simulink model "ZT_VehCtrl_18B"  (R2018b)
settings: Solver=FixedStepAuto  StartTime=0.0  StopTime=inf  FixedStep=0.005  RelTol=1e-3
InitFcn:
  | mbd_mpc_consistency_checks(bdroot(gcs));
undefined symbols (not defined in the file): ANG_DEAD, BMS_NormalPwr, BrkPrsByBrkPct_TB_X, BrkPrsByBrkPct_TB_Y, DELAY_DISCHARGE, DELAY_RCUOFF, DRV_BACKWARD, DRV_BRAKE, DRV_FORWARD, DRV_NEUTRAL, DRV_PARK, DRV_UNPARK, DRV_ZEROTURN, EPB_LOCK, EPB_UNLOCK, ExtraLoadPwr, FanOff, fifo_0_vect, fifo_1_vect, HiFanReq, HV_finished, HV_No_Active, HV_POWER_OFF, HV_POWER_ON, HVDown, HVON, KaTLS_v_DrgUp_X_VehSpd, KeFTM_s_Way1OffDlyTime, KeFTM_TK_Way1CoolLv2OffBatTemp, KeFTM_TK_Way1CoolLv2OffMtrTemp, KeFTM_TK_Way1CoolLv2OnBatTemp, KeFTM_TK_Way1CoolLv2OnMtrTemp, KeFTM_TK_Way1CoolLv3OffBatTemp, KeFTM_TK_Way1CoolLv3OffMtrTemp, KeFTM_TK_Way1CoolLv3OnBatTemp, KeFTM_TK_Way1CoolLv3OnMtrTemp, KeFTM_TK_Way1CoolLv4OffBatTemp, KeFTM_TK_Way1CoolLv4OffMtrTemp, KeFTM_TK_Way1CoolLv4OnBatTemp, KeFTM_TK_Way1CoolLv4OnMtrTemp, Kp1, Kp2, LowFanReq, LQFP, MtrPwrFactor_RCU, MtrPwrHighToMidThd, MtrPwrLowToMidThd, MtrPwrMidToHighThd, MtrPwrMidToLowThd, MtrTrqMax, PCT_DEAD, Precharge, PTO_1000, PTO_540, pts1_fifo_0_vect, pts1_fifo_1_vect, pts2_fifo_0_vect, pts2_fifo_1_vect, pts3_fifo_0_vect, pts3_fifo_1_vect ... (+24)
libraries: mbd_mpc574x_ec_toolbox x124, canmsglib x72, simulink x57
(part 4 of 11)

== system ZT_VehCtrl_18B/VehCtrl/EnergyManage1 ==
  DriverIn : Inport
  VehTrqTgt : Inport  Port=2
  VehSpd : Inport  Port=3
  RCU : Inport  Port=4
  Fault : Inport  Port=5
  MCU_PTO : Inport  Port=6
  BMS : Inport  Port=7
  "RMT " : Inport  Port=8
  MtrPwrOutTotal : Inport  Port=9
  Add : Sum
  Bus Creator1 : BusCreator  Inputs=7
  Bus Creator2 : BusCreator  Inputs=2
  Bus Creator3 : BusCreator  Inputs=1
  Bus Creator4 : BusCreator  Inputs=1
  Bus Selector : BusSelector  OutputSignals=KeyStatus
  Bus Selector1 : BusSelector  OutputSignals=ShutDown
  Bus Selector2 : BusSelector  OutputSignals=OBC_Charger Status.RCU_RexSelfChkSt,OBC_Charger Status.RCU_RexFltLvl,BMS_Charger Status.RCU_RexGenPwrMaxLim,RCU_MSG_3.RCU_GCUISGInverterTempHiAlarm,RCU_MSG_3.RCU_GCUISGMotorTempHiAlarm
  Bus Selector3 : BusSelector  OutputSignals=RMT4.RMT_RCU
  Bus Selector4 : BusSelector  OutputSignals=BMS Power Infor.APPSOC,BMS_PackStateInf.BMS_BatteryState,BMS_Relay Status.IPI_ChrgSignal,BMS_Relay Status.IPI_CC2St
  Chart : Stateflow chart  TreatAsAtomicUnit=on
  Chart1 : Stateflow chart  TreatAsAtomicUnit=on
  Constant : Constant  Value=ExtraLoadPwr
  Data Store Write : DataStoreWrite  DataStoreName=Flag
  Logical Operator : Logic  Operator=OR  AllPortsSameDT=off  OutDataTypeStr=boolean
  Subsystem : Subsystem
  BMS_OUT : Outport
  RCU_OUT : Outport  Port=2
  DCDC_OUT : Outport  Port=3
  MCU_COM : Outport  Port=4
  Ready : Outport  Port=5
  EN_COM : Outport  Port=6
  wires:
  Add/1 -> Chart1/1(MtrPwrTotal)
  Chart/7(VCU_MotwaterPumpDutyRe) -> Bus Creator1/6  "VCU_MotwaterPumpDutyRe"
  Constant/1 -> Add/2
  MtrPwrOutTotal/1 -> Add/1
  Chart1/1(RCU_RexGenPwr) -> Chart/13(RCU_RexGenPwr)
  Bus Selector4/1 -> Chart/9(BMS_SOC)  "<APPSOC>"
  Bus Selector2/1 -> Chart/3(RCU_RexSelfChkSt)  "<RCU_RexSelfChkSt>"
  Chart/13(Flag) -> Data Store Write/1
  Chart/1(VCU_Maincircuitcommand) -> Bus Creator4/1  "VCU_Maincircuitcommand"
  Chart/3(VCU_RexEnableCmd) -> Bus Creator1/2  "VCU_RexEnableCmd"
  "RMT "/1 -> Bus Selector3/1
  VehSpd/1 -> Subsystem/2(VehSpd)
  Bus Creator2/1 -> MCU_COM/1
  Bus Selector4/3 -> Logical Operator/1  "<IPI_ChrgSignal>"
  Chart/8(VCU_RexActiveDischgCmd) -> Bus Creator1/7  "VCU_RexActiveDischgCmd"
  VehTrqTgt/1 -> Subsystem/1(VehTrqTgt)
  Bus Selector3/1 -> Chart/12(Rcuswitch)  "<RMT_RCU>"
  Bus Selector4/4 -> Logical Operator/2  "<IPI_CC2St>"
  Chart/11(Ready) -> Ready/1  "Ready"
  Bus Selector2/5 -> Chart/7(RCU_GCUISGMotorTempHiAlarm)  "<RCU_GCUISGMotorTempHiAlarm>"
  Chart/6(VCU_FanStsReg) -> Bus Creator1/5  "VCU_FanStsReg"
  Bus Selector2/4 -> Chart/6(RCU_GCUISGInverterTempHiAlarm)  "<RCU_GCUISGInverterTempHiAlarm>"
  Bus Creator3/1 -> DCDC_OUT/1
  Bus Creator4/1 -> BMS_OUT/1
  Bus Selector/1 -> Chart/1(Key)  "<KeyStatus>"
  Chart/12(DCDC_Enable) -> Bus Creator3/1  "DCDC_Enable"
  Chart/10(MCU_Discharge) -> Bus Creator2/2  "MCU_Discharge"
  Bus Selector2/3 -> Chart/5(RCU_RexGenPwrMaxLim)  "<RCU_RexGenPwrMaxLim>"
  Chart/4(VCU_RexStartStopReq) -> Bus Creator1/3  "VCU_RexStartStopReq"
  Bus Creator1/1 -> RCU_OUT/1
  Subsystem/1(PwrCmd) -> Chart/8(MCU_TotalPwrCmd)
  Chart/2(VCU_HVOnOffSts) -> Bus Creator1/1  "VCU_HVOnOffSts"
  DriverIn/1 -> Bus Selector/1
  RCU/1 -> Bus Selector2/1
  Bus Selector2/2 -> Chart/4(RCU_RexFltLvl)  "<RCU_RexFltLvl>"
  Bus Selector4/2 -> Chart/10(BMS_BatteryState)  "<BMS_BatteryState>"
  Fault/1 -> Bus Selector1/1
  BMS/1 -> Bus Selector4/1
  MCU_PTO/1 -> Subsystem/3(MCU_PTO)
  Chart/5(VCU_ReqRexGenPwr) -> Bus Creator1/4  "VCU_ReqRexGenPwr"
  Logical Operator/1 -> Chart/11(ChrgSig)
  Chart/9(MCU_Enable) -> Bus Creator2/1, EN_COM/1  "MCU_Enable"
  Bus Selector1/1 -> Chart/2(ShutDown)  "<ShutDown>"

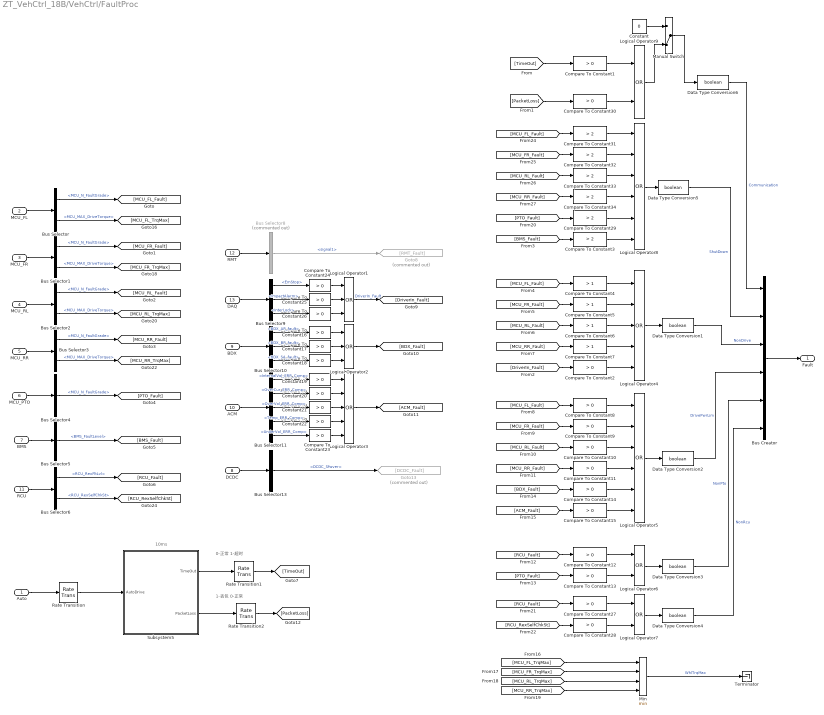
== system ZT_VehCtrl_18B/VehCtrl/FaultProc ==
  note: 10ms
  note: 0-正常
      | 1-超时
  note: 1-丢包
      | 0-正常
  Auto : Inport
  MCU_FL : Inport  Port=2
  MCU_FR : Inport  Port=3
  MCU_RL : Inport  Port=4
  MCU_RR : Inport  Port=5
  MCU_PTO : Inport  Port=6
  BMS : Inport  Port=7
  DCDC : Inport  Port=8
  BDX : Inport  Port=9
  ACM : Inport  Port=10
  RCU : Inport  Port=11
  RMT : Inport  Port=12
  DAQ : Inport  Port=13
  Bus Creator : BusCreator  Inputs=6
  Bus Selector{,1..3} (4 alike) : BusSelector  OutputSignals=MCU2VCU_3.MCU_N_FaultGrade,MCU2VCU_4.MCU_MAX_DriveTorque
  Bus Selector10 : BusSelector  OutputSignals=AVCU.BDX_AP_fault,AVCU.BDX_BP_fault,AVCU.BDX_SA_fault
  Bus Selector11 : BusSelector  OutputSignals=InternalVol_ERR_Comp,OverCur_ERR_Comp,OverVol_ERR_Comp,Temp_ERR_Comp,UnderVol_ERR_Comp
  Bus Selector13 : BusSelector  OutputSignals=DCDC_Sfwver
  Bus Selector4 : BusSelector  OutputSignals=MCU2VCU_3.MCU_N_FaultGrade
  Bus Selector5 : BusSelector  OutputSignals=BMS_PackStateInf.BMS_FaultLevel
  Bus Selector6 : BusSelector  OutputSignals=OBC_Charger Status.RCU_RexFltLvl,OBC_Charger Status.RCU_RexSelfChkSt
  Bus Selector8 : BusSelector  Commented=on  OutputSignals=RMT3.signal1
  Bus Selector9 : BusSelector  OutputSignals=EmStop,ImpactAlarm,InterLock
  Compare To Constant{1..2,8..28,30} (24 alike) : simulink/Logic and Bit Operations/Compare To Constant  relop=>  const=0  OutDataTypeStr=boolean
  Compare To Constant{3,29,31..34} (6 alike) : simulink/Logic and Bit Operations/Compare To Constant  relop=>  const=2  OutDataTypeStr=boolean
  Compare To Constant{4..7} (4 alike) : simulink/Logic and Bit Operations/Compare To Constant  relop=>  const=1  OutDataTypeStr=boolean
  Constant : Constant  Value=0
  Data Type Conversion{1..6} (6 alike) : DataTypeConversion  OutDataTypeStr=boolean
  Goto13 : Goto  Commented=on  GotoTag=DCDC_Fault
  Goto8 : Goto  Commented=on  GotoTag=RMT_Fault
  Logical Operator1 : Logic  Operator=OR  Inputs=3  AllPortsSameDT=off  OutDataTypeStr=boolean
  Logical Operator2 : Logic  Operator=OR  Inputs=3  AllPortsSameDT=off  OutDataTypeStr=boolean
  Logical Operator3 : Logic  Operator=OR  Inputs=5  AllPortsSameDT=off  OutDataTypeStr=boolean
  Logical Operator4 : Logic  Operator=OR  Inputs=5  AllPortsSameDT=off  OutDataTypeStr=boolean
  Logical Operator5 : Logic  Operator=OR  Inputs=6  AllPortsSameDT=off  OutDataTypeStr=boolean
  Logical Operator6 : Logic  Operator=OR  AllPortsSameDT=off  OutDataTypeStr=boolean
  Logical Operator7 : Logic  Operator=OR  AllPortsSameDT=off  OutDataTypeStr=boolean
  Logical Operator8 : Logic  Operator=OR  Inputs=6  AllPortsSameDT=off  OutDataTypeStr=boolean
  Logical Operator9 : Logic  Operator=OR  AllPortsSameDT=off  OutDataTypeStr=boolean
  Manual Switch : ManualSwitch  CurrentSetting=0
  Min : MinMax  Inputs=4
  Rate Transition : RateTransition
  Rate Transition1 : RateTransition
  Rate Transition2 : RateTransition
  Subsystem5 : Subsystem  TreatAsAtomicUnit=on  SystemSampleTime=0.01
  Terminator : Terminator
  Fault : Outport
  wires:
  Logical Operator8/1 -> Data Type Conversion5/1
  Data Type Conversion1/1 -> Bus Creator/3  "NonDrive"
  Data Type Conversion2/1 -> Bus Creator/4  "DrivePwrLim"
  Data Type Conversion3/1 -> Bus Creator/5  "NonPto"
  Bus Creator/1 -> Fault/1
  MCU_FL/1 -> Bus Selector/1
  Bus Selector/1 -> [MCU_FL_Fault]  "<MCU_N_FaultGrade>"
  Bus Selector1/1 -> [MCU_FR_Fault]  "<MCU_N_FaultGrade>"
  MCU_FR/1 -> Bus Selector1/1
  MCU_RR/1 -> Bus Selector3/1
  Bus Selector3/1 -> [MCU_RR_Fault]  "<MCU_N_FaultGrade>"
  Bus Selector2/1 -> [MCU_RL_Fault]  "<MCU_N_FaultGrade>"
  MCU_RL/1 -> Bus Selector2/1
  Bus Selector4/1 -> [PTO_Fault]  "<MCU_N_FaultGrade>"
  MCU_PTO/1 -> Bus Selector4/1
  BMS/1 -> Bus Selector5/1
  Bus Selector5/1 -> [BMS_Fault]  "<BMS_FaultLevel>"
  Bus Selector6/1 -> [RCU_Fault]  "<RCU_RexFltLvl>"
  RCU/1 -> Bus Selector6/1
  Bus Selector8/1 -> Goto8/1  "<signal1>"
  RMT/1 -> Bus Selector8/1
  DAQ/1 -> Bus Selector9/1
  Bus Selector9/1 -> Compare To Constant24/1  "<EmStop>"
  Bus Selector9/2 -> Compare To Constant25/1  "<ImpactAlarm>"
  Bus Selector9/3 -> Compare To Constant26/1  "<InterLock>"
  Logical Operator1/1 -> [DriverIn_Fault]  "DriverIn_Fault"
  BDX/1 -> Bus Selector10/1
  Logical Operator2/1 -> [BDX_Fault]
  Bus Selector10/3 -> Compare To Constant18/1  "<BDX_SA_fault>"
  Bus Selector10/2 -> Compare To Constant17/1  "<BDX_BP_fault>"
  Bus Selector10/1 -> Compare To Constant16/1  "<BDX_AP_fault>"
  ACM/1 -> Bus Selector11/1
  Bus Selector11/1 -> Compare To Constant19/1  "<InternalVol_ERR_Comp>"
  Bus Selector11/2 -> Compare To Constant20/1  "<OverCur_ERR_Comp>"
  Bus Selector11/3 -> Compare To Constant21/1  "<OverVol_ERR_Comp>"
  Logical Operator3/1 -> [ACM_Fault]
  Bus Selector11/4 -> Compare To Constant22/1  "<Temp_ERR_Comp>"
  Bus Selector11/5 -> Compare To Constant23/1  "<UnderVol_ERR_Comp>"
  DCDC/1 -> Bus Selector13/1
  Bus Selector13/1 -> Goto13/1  "<DCDC_Sfwver>"
  [DriverIn_Fault] -> Compare To Constant2/1
  [BMS_Fault] -> Compare To Constant3/1
  Logical Operator4/1 -> Data Type Conversion1/1
  [MCU_FL_Fault] -> Compare To Constant4/1
  Compare To Constant4/1 -> Logical Operator4/1
  Compare To Constant5/1 -> Logical Operator4/2
  [MCU_FR_Fault] -> Compare To Constant5/1
  [MCU_RR_Fault] -> Compare To Constant7/1
  Compare To Constant7/1 -> Logical Operator4/4
  Compare To Constant6/1 -> Logical Operator4/3
  [MCU_RL_Fault] -> Compare To Constant6/1
  Logical Operator5/1 -> Data Type Conversion2/1
  [MCU_RL_Fault] -> Compare To Constant10/1
  Compare To Constant10/1 -> Logical Operator5/3
  Compare To Constant11/1 -> Logical Operator5/4
  [MCU_RR_Fault] -> Compare To Constant11/1
  [MCU_FR_Fault] -> Compare To Constant9/1
  Compare To Constant9/1 -> Logical Operator5/2
  Compare To Constant8/1 -> Logical Operator5/1
  [MCU_FL_Fault] -> Compare To Constant8/1
  Logical Operator6/1 -> Data Type Conversion3/1
  [RCU_Fault] -> Compare To Constant12/1
  Compare To Constant12/1 -> Logical Operator6/1
  Compare To Constant13/1 -> Logical Operator6/2
  [PTO_Fault] -> Compare To Constant13/1
  [BDX_Fault] -> Compare To Constant14/1
  Compare To Constant14/1 -> Logical Operator5/5
  Compare To Constant15/1 -> Logical Operator5/6
  [ACM_Fault] -> Compare To Constant15/1
  Bus Selector/2 -> [MCU_FL_TrqMax]  "<MCU_MAX_DriveTorque>"
  Bus Selector1/2 -> [MCU_FR_TrqMax]  "<MCU_MAX_DriveTorque>"
  Bus Selector2/2 -> [MCU_RL_TrqMax]  "<MCU_MAX_DriveTorque>"
  Bus Selector3/2 -> [MCU_RR_TrqMax]  "<MCU_MAX_DriveTorque>"
  [MCU_FL_TrqMax] -> Min/1
  [MCU_FR_TrqMax] -> Min/2
  [MCU_RL_TrqMax] -> Min/3
  [MCU_RR_TrqMax] -> Min/4
  Compare To Constant16/1 -> Logical Operator2/1
  Compare To Constant17/1 -> Logical Operator2/2
  Compare To Constant18/1 -> Logical Operator2/3
  Compare To Constant19/1 -> Logical Operator3/1
  Compare To Constant20/1 -> Logical Operator3/2
  Compare To Constant21/1 -> Logical Operator3/3
  Compare To Constant22/1 -> Logical Operator3/4
  Compare To Constant23/1 -> Logical Operator3/5
  Compare To Constant24/1 -> Logical Operator1/1
  Compare To Constant25/1 -> Logical Operator1/2
  Compare To Constant26/1 -> Logical Operator1/3
  Bus Selector6/2 -> [RCU_RexSelfChkSt]  "<RCU_RexSelfChkSt>"
  [RCU_RexSelfChkSt] -> Compare To Constant28/1
  Compare To Constant28/1 -> Logical Operator7/2
  Compare To Constant27/1 -> Logical Operator7/1
  [RCU_Fault] -> Compare To Constant27/1
  Logical Operator7/1 -> Data Type Conversion4/1
  Data Type Conversion4/1 -> Bus Creator/6  "NonRcu"
  Compare To Constant2/1 -> Logical Operator4/5
  [MCU_RL_Fault] -> Compare To Constant33/1
  Compare To Constant33/1 -> Logical Operator8/3
  Compare To Constant34/1 -> Logical Operator8/4
  [MCU_RR_Fault] -> Compare To Constant34/1
  [MCU_FR_Fault] -> Compare To Constant32/1
  Compare To Constant32/1 -> Logical Operator8/2
  Compare To Constant31/1 -> Logical Operator8/1
  [MCU_FL_Fault] -> Compare To Constant31/1
  Compare To Constant3/1 -> Logical Operator8/6
  [PTO_Fault] -> Compare To Constant29/1
  Compare To Constant29/1 -> Logical Operator8/5
  Min/1 -> Terminator/1  "WhlTrqMax"
  Rate Transition1/1 -> [TimeOut]
  Auto/1 -> Rate Transition/1
  Subsystem5/2(PacketLoss) -> Rate Transition2/1
  Rate Transition/1 -> Subsystem5/1(AutoDrive)
  Rate Transition2/1 -> [PacketLoss]
  Subsystem5/1(TimeOut) -> Rate Transition1/1
  Data Type Conversion5/1 -> Bus Creator/2  "ShutDown"
  [TimeOut] -> Compare To Constant1/1
  [PacketLoss] -> Compare To Constant30/1
  Compare To Constant1/1 -> Logical Operator9/1
  Compare To Constant30/1 -> Logical Operator9/2
  Manual Switch/1 -> Data Type Conversion6/1
  Data Type Conversion6/1 -> Bus Creator/1  "Communication"
  Constant/1 -> Manual Switch/1
  Logical Operator9/1 -> Manual Switch/2

== system ZT_VehCtrl_18B/VehCtrl/LedControl ==
  note: LS015-红灯
      | LS016-绿灯
      | 都亮为黄灯
  BMS : Inport
  cmd : Inport  Port=2
  Bus Selector : BusSelector  OutputSignals=StrAng,BrkPct,ModeDir
  Bus Selector1 : BusSelector  OutputSignals=BMS_PackStateInf.BMS_BatteryState,BMS Power Infor.APPSOC
  Chart : Stateflow chart  TreatAsAtomicUnit=on
  Chart1 : Stateflow chart  TreatAsAtomicUnit=on
  Compare To Constant : simulink/Logic and Bit Operations/Compare To Constant  relop===  const=3.0  OutDataTypeStr=boolean
  Constant : Constant  Value=0  OutDataTypeStr=boolean
  Constant1 : Constant  OutDataTypeStr=boolean
  Data Store Read : DataStoreRead  DataStoreName=Fault
  Data Store Read1 : DataStoreRead  DataStoreName=CtrMode
  Data Store Write : DataStoreWrite  DataStoreName=HS002
  Data Store Write1 : DataStoreWrite  DataStoreName=HS003
  Data Store Write2 : DataStoreWrite  DataStoreName=HS005
  Data Store Write3 : DataStoreWrite  DataStoreName=HS007
  Data Store Write4 : DataStoreWrite  DataStoreName=HS010
  Data Store Write5 : DataStoreWrite  DataStoreName=LS015
  Data Store Write6 : DataStoreWrite  DataStoreName=LS016
  Data Type Conversion{,1..3} (4 alike) : DataTypeConversion  OutDataTypeStr=boolean
  Data Type Conversion{4..7} (4 alike) : DataTypeConversion
  Switch : Switch  Threshold=1
  wires:
  cmd/1 -> Bus Selector/1
  Bus Selector/1 -> Chart/2(SteerAng)  "<StrAng>"
  Chart/1(Left_Cmd) -> Data Type Conversion1/1
  Chart/2(Right_Cmd) -> Data Type Conversion2/1
  Bus Selector/2 -> Switch/2  "<BrkPct>"
  Bus Selector/3 -> Data Type Conversion/1  "<ModeDir>"
  Data Type Conversion1/1 -> Data Store Write1/1
  Data Type Conversion2/1 -> Data Store Write/1
  Switch/1 -> Data Store Write3/1
  Data Type Conversion/1 -> Data Store Write4/1
  Constant1/1 -> Switch/1
  Constant/1 -> Switch/3
  BMS/1 -> Bus Selector1/1
  Bus Selector1/2 -> Chart/1(soc)  "<APPSOC>"
  Data Type Conversion3/1 -> Data Store Write2/1
  Compare To Constant/1 -> Data Type Conversion3/1
  Bus Selector1/1 -> Compare To Constant/1  "<BMS_BatteryState>"
  Chart1/1(Red) -> Data Type Conversion4/1
  Chart1/2(Green) -> Data Type Conversion5/1
  Data Store Read1/1 -> Data Type Conversion6/1
  Data Store Read/1 -> Data Type Conversion7/1
  Data Type Conversion4/1 -> Data Store Write5/1
  Data Type Conversion5/1 -> Data Store Write6/1
  Data Type Conversion6/1 -> Chart1/1(CtrMode)
  Data Type Conversion7/1 -> Chart1/2(Fault)

== system ZT_VehCtrl_18B/VehCtrl/MontionControl ==
  EN_COM : Inport
  Ready : Inport  Port=2
  CMD : Inport  Port=3
  VehSpd : Inport  Port=4
  BDX : Inport  Port=5
  Fault : Inport  Port=6
  AUTOMode : Inport  Port=7
  AUTO : Inport  Port=8
  BMS : Inport  Port=9
  RMT : Inport  Port=10
  DCDC : Inport  Port=11
  DriveControl : Subsystem
  PtoControl : Subsystem
  SteerControl : Subsystem
  ValveControl : Subsystem
  MCUFL_OUT : Outport
  MCUFR_OUT : Outport  Port=2
  MCURL_OUT : Outport  Port=3
  MCURR_OUT : Outport  Port=4
  MCU_PTO_OUT : Outport  Port=5
  BDX_OUT : Outport  Port=6
  VehTrqTgt : Outport  Port=7
  wires:
  CMD/1 -> PtoControl/1(CMD), ValveControl/4(CMD), SteerControl/2(CMD), DriveControl/4(CMD)
  BDX/1 -> ValveControl/3(BDX), SteerControl/3(BDX)
  SteerControl/1(StrReady) -> DriveControl/7(StrReady)
  VehSpd/1 -> ValveControl/8(VehSpd), SteerControl/1(VehSpd), DriveControl/6(VehSpd)
  DriveControl/5(BrkPrsTgt) -> ValveControl/1(BrkPrsTgt)
  DriveControl/6(EpbSt) -> ValveControl/2(EpbSt)
  DriveControl/1(MCUFL_OUT) -> MCUFL_OUT/1
  DriveControl/2(MCUFR_OUT) -> MCUFR_OUT/1
  DriveControl/4(MCURR_OUT) -> MCURR_OUT/1
  DriveControl/3(MCURL_OUT) -> MCURL_OUT/1
  ValveControl/1(BDX_OUT) -> BDX_OUT/1
  Ready/1 -> PtoControl/3(Ready), ValveControl/5(Ready), DriveControl/2(Ready)
  PtoControl/1(MCU_PTO_OUT) -> MCU_PTO_OUT/1
  DriveControl/7(VehTrqTgt) -> VehTrqTgt/1
  SteerControl/2(AngCmd) -> ValveControl/6("AngCmd ")
  AUTOMode/1 -> PtoControl/4(AUTOMode), DriveControl/9(AUTOMode)
  AUTO/1 -> PtoControl/5(AUTO), DriveControl/8(AUTO)
  BMS/1 -> DriveControl/5(BMS)
  RMT/1 -> DriveControl/10(RMT)
  DCDC/1 -> DriveControl/11(DCDC)
  Fault/1 -> PtoControl/2(Fault), ValveControl/7(fault), DriveControl/3(Fault)
  EN_COM/1 -> DriveControl/1(EN_COM)

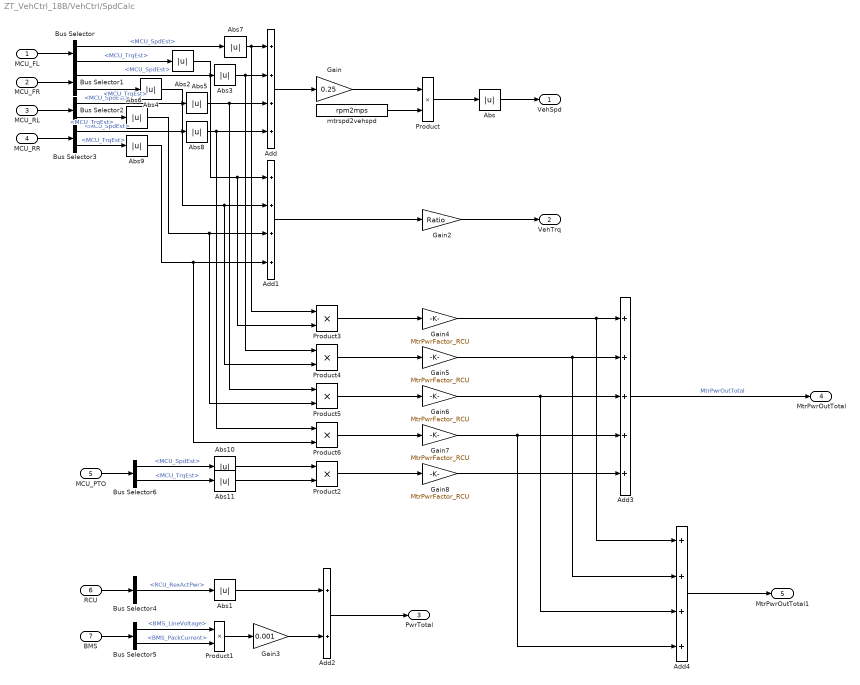
== system ZT_VehCtrl_18B/VehCtrl/SpdCalc ==
  MCU_FL : Inport
  MCU_FR : Inport  Port=2
  MCU_RL : Inport  Port=3
  MCU_RR : Inport  Port=4
  MCU_PTO : Inport  Port=5
  RCU : Inport  Port=6
  BMS : Inport  Port=7
  Abs{,1..11} (12 alike) : Abs
  Add : Sum  Inputs=++++
  Add1 : Sum  Inputs=++++
  Add2 : Sum
  Add3 : Sum  Inputs=+++++
  Add4 : Sum  Inputs=4
  Bus Selector{,1..3,6} (5 alike) : BusSelector  OutputSignals=MCU2VCU_1.MCU_SpdEst,MCU2VCU_1.MCU_TrqEst
  Bus Selector4 : BusSelector  OutputSignals=BMS_Charger Status.RCU_RexActPwr
  Bus Selector5 : BusSelector  OutputSignals=BMS_PackMeasure.BMS_LineVoltage,BMS_PackMeasure.BMS_PackCurrent
  Gain : Gain  Gain=0.25
  Gain2 : Gain  Gain=Ratio
  Gain3 : Gain  Gain=0.001
  Gain{4..8} (5 alike) : Gain  Gain=MtrPwrFactor_RCU
  Product{,1..6} (7 alike) : Product
  mtrspd2vehspd : Constant  Value=rpm2mps
  VehSpd : Outport
  "VehTrq " : Outport  Port=2
  PwrTotal : Outport  Port=3
  MtrPwrOutTotal : Outport  Port=4
  MtrPwrOutTotal1 : Outport  Port=5
  wires:
  Add/1 -> Gain/1
  Gain/1 -> Product/1
  Product/1 -> Abs/1
  mtrspd2vehspd/1 -> Product/2
  MCU_FL/1 -> Bus Selector/1
  Bus Selector/1 -> Abs7/1  "<MCU_SpdEst>"
  Bus Selector1/1 -> Abs3/1  "<MCU_SpdEst>"
  MCU_FR/1 -> Bus Selector1/1
  MCU_RR/1 -> Bus Selector3/1
  Bus Selector3/1 -> Abs8/1  "<MCU_SpdEst>"
  Bus Selector2/1 -> Abs5/1  "<MCU_SpdEst>"
  MCU_RL/1 -> Bus Selector2/1
  Abs/1 -> VehSpd/1
  Bus Selector/2 -> Abs2/1  "<MCU_TrqEst>"
  Bus Selector1/2 -> Abs4/1  "<MCU_TrqEst>"
  Bus Selector2/2 -> Abs6/1  "<MCU_TrqEst>"
  Bus Selector3/2 -> Abs9/1  "<MCU_TrqEst>"
  Add1/1 -> Gain2/1
  Gain2/1 -> "VehTrq "/1
  RCU/1 -> Bus Selector4/1
  BMS/1 -> Bus Selector5/1
  Bus Selector5/1 -> Product1/1  "<BMS_LineVoltage>"
  Bus Selector5/2 -> Product1/2  "<BMS_PackCurrent>"
  Product1/1 -> Gain3/1
  Bus Selector4/1 -> Abs1/1  "<RCU_RexActPwr>"
  Gain3/1 -> Add2/2
  Abs1/1 -> Add2/1
  Add2/1 -> PwrTotal/1
  MCU_PTO/1 -> Bus Selector6/1
  Bus Selector6/1 -> Abs10/1  "<MCU_SpdEst>"
  Bus Selector6/2 -> Abs11/1  "<MCU_TrqEst>"
  Product3/1 -> Gain4/1
  Product2/1 -> Gain8/1
  Product6/1 -> Gain7/1
  Product5/1 -> Gain6/1
  Product4/1 -> Gain5/1
  Gain4/1 -> Add4/1, Add3/1
  Gain5/1 -> Add4/2, Add3/2
  Gain6/1 -> Add4/3, Add3/3
  Gain8/1 -> Add3/5
  Add3/1 -> MtrPwrOutTotal/1  "MtrPwrOutTotal"
  Gain7/1 -> Add4/4, Add3/4
  Abs7/1 -> Product3/1, Add/1
  Abs2/1 -> Product3/2, Add1/1
  Abs3/1 -> Product4/1, Add/2
  Abs4/1 -> Product4/2, Add1/2
  Abs5/1 -> Product5/1, Add/3
  Abs6/1 -> Product5/2, Add1/3
  Abs8/1 -> Product6/1, Add/4
  Abs9/1 -> Product6/2, Add1/4
  Abs10/1 -> Product2/1
  Abs11/1 -> Product2/2
  Add4/1 -> MtrPwrOutTotal1/1

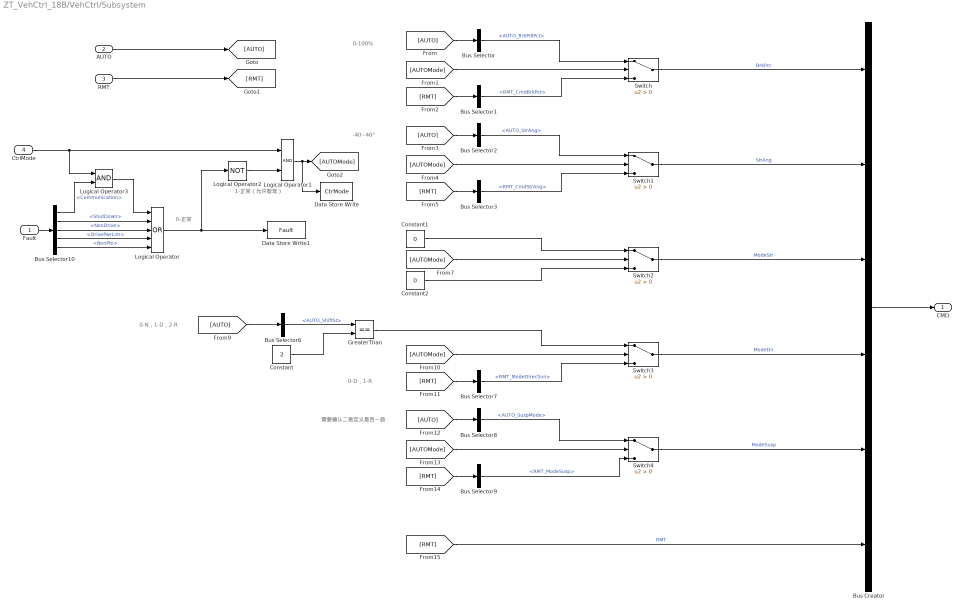
== system ZT_VehCtrl_18B/VehCtrl/Subsystem ==
  note: 0-正常
  note: -40~40°
  note: 0-100%
  note: 0-N，1-D，2-R
  note: 0-D，1-R
  note: 需要确认二者定义是否一致
  note: 1-正常（允许智驾）
  Fault : Inport
  AUTO : Inport  Port=2
  RMT : Inport  Port=3
  CtrlMode : Inport  Port=4
  Bus Creator : BusCreator  Inputs=6
  Bus Selector : BusSelector  OutputSignals=signal1.AUTO_BrkPdlPct
  Bus Selector1 : BusSelector  OutputSignals=RMT1.RMT_CmdBrkPct
  Bus Selector10 : BusSelector  OutputSignals=Communication,ShutDown,NonDrive,DrivePwrLim,NonPto
  Bus Selector2 : BusSelector  OutputSignals=signal1.AUTO_StrAng
  Bus Selector3 : BusSelector  OutputSignals=RMT1.RMT_CmdStrAng
  Bus Selector6 : BusSelector  OutputSignals=signal1.AUTO_ShiftSt
  Bus Selector7 : BusSelector  OutputSignals=RMT3.RMT_ModeDirection
  Bus Selector8 : BusSelector  OutputSignals=signal2.AUTO_SuspMode
  Bus Selector9 : BusSelector  OutputSignals=RMT2.RMT_ModeSusp
  Constant : Constant  Value=2  OutDataTypeStr=uint8
  Constant1 : Constant  Value=0  OutDataTypeStr=boolean
  Constant2 : Constant  Value=0  OutDataTypeStr=boolean
  Data Store Write : DataStoreWrite  DataStoreName=CtrMode
  Data Store Write1 : DataStoreWrite  DataStoreName=Fault
  GreaterThan : RelationalOperator  Operator===  OutDataTypeStr=boolean  RndMeth=Simplest
  Logical Operator : Logic  Operator=OR  Inputs=5  AllPortsSameDT=off  OutDataTypeStr=boolean
  Logical Operator1 : Logic  AllPortsSameDT=off  OutDataTypeStr=boolean
  Logical Operator2 : Logic  Operator=NOT  AllPortsSameDT=off  OutDataTypeStr=boolean
  Logical Operator3 : Logic  AllPortsSameDT=off  OutDataTypeStr=boolean
  Switch{,1..4} (5 alike) : Switch  Criteria=u2 > Threshold
  CMD : Outport
  wires:
  Switch/1 -> Bus Creator/1  "BrkPct"
  Bus Selector/1 -> Switch/1  "<AUTO_BrkPdlPct>"
  Bus Selector1/1 -> Switch/3  "<RMT_CmdBrkPct>"
  AUTO/1 -> [AUTO]
  RMT/1 -> [RMT]
  [AUTO] -> Bus Selector/1
  [RMT] -> Bus Selector1/1
  [AUTOMode] -> Switch/2
  [RMT] -> Bus Selector3/1
  [AUTO] -> Bus Selector2/1
  Bus Selector2/1 -> Switch1/1  "<AUTO_StrAng>"
  [AUTOMode] -> Switch1/2
  Bus Selector3/1 -> Switch1/3  "<RMT_CmdStrAng>"
  Switch1/1 -> Bus Creator/2  "StrAng"
  [AUTOMode] -> Switch2/2
  Switch2/1 -> Bus Creator/3  "ModeStr"
  [RMT] -> Bus Selector7/1
  [AUTO] -> Bus Selector6/1
  [AUTOMode] -> Switch3/2
  Bus Selector7/1 -> Switch3/3  "<RMT_ModeDirection>"
  Switch3/1 -> Bus Creator/4  "ModeDir"
  [RMT] -> Bus Selector9/1
  [AUTO] -> Bus Selector8/1
  Bus Selector8/1 -> Switch4/1  "<AUTO_SuspMode>"
  [AUTOMode] -> Switch4/2
  Bus Selector9/1 -> Switch4/3  "<RMT_ModeSusp>"
  Switch4/1 -> Bus Creator/5  "ModeSusp"
  Bus Creator/1 -> CMD/1
  [RMT] -> Bus Creator/6  "RMT"
  CtrlMode/1 -> Logical Operator3/1, Logical Operator1/1
  Bus Selector6/1 -> GreaterThan/1  "<AUTO_ShiftSt>"
  GreaterThan/1 -> Switch3/1
  Constant/1 -> GreaterThan/2
  Logical Operator/1 -> Logical Operator2/1, Data Store Write1/1
  Logical Operator2/1 -> Logical Operator1/2
  Logical Operator1/1 -> Data Store Write/1, [AUTOMode]
  Fault/1 -> Bus Selector10/1
  Bus Selector10/1 -> Logical Operator3/2  "<Communication>"
  Bus Selector10/2 -> Logical Operator/2  "<ShutDown>"
  Bus Selector10/3 -> Logical Operator/3  "<NonDrive>"
  Bus Selector10/4 -> Logical Operator/4  "<DrivePwrLim>"
  Bus Selector10/5 -> Logical Operator/5  "<NonPto>"
  Logical Operator3/1 -> Logical Operator/1
  Constant1/1 -> Switch2/1
  Constant2/1 -> Switch2/3

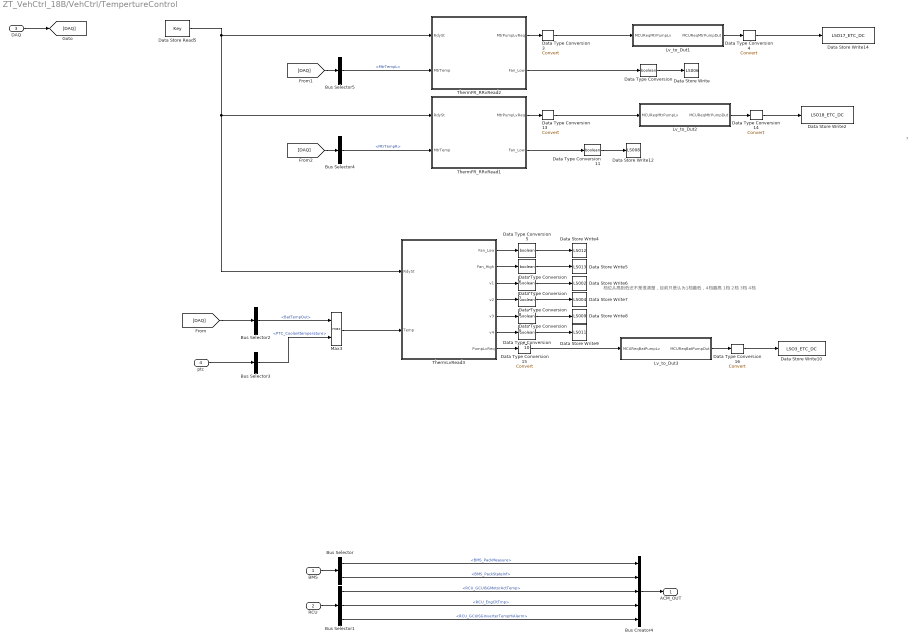
== system ZT_VehCtrl_18B/VehCtrl/TempertureControl ==
  note: 档位从高到低还不是很清楚，目前只是认为1档最低，4档最高
      | 1档
      | 2档
      | 3档
      | 4档
  note: ?
  BMS : Inport
  RCU : Inport  Port=2
  DAQ : Inport  Port=3
  ptc : Inport  Port=4
  Bus Creator4 : BusCreator  Inputs=5
  Bus Selector : BusSelector  OutputSignals=BMS_PackMeasure,BMS_PackStateInf
  Bus Selector1 : BusSelector  OutputSignals=RCU_MSG_3.RCU_GCUISGMotorActTemp,RCU_MSG_3.RCU_EngCltTmp,RCU_MSG_3.RCU_GCUISGInverterTempHiAlarm
  Bus Selector2 : BusSelector  OutputSignals=BatTempOut
  Bus Selector3 : BusSelector  OutputSignals=signal1.PTC_Coolanttemperature
  Bus Selector4 : BusSelector  OutputSignals=MtrTempR
  Bus Selector5 : BusSelector  OutputSignals=MtrTempL
  Data Store Read5 : DataStoreRead  DataStoreName=Key
  Data Store Write : DataStoreWrite  DataStoreName=LS006
  Data Store Write10 : DataStoreWrite  DataStoreName=LSO3_ETC_DC
  Data Store Write12 : DataStoreWrite  DataStoreName=LS008
  Data Store Write14 : DataStoreWrite  DataStoreName=LSO17_ETC_DC
  Data Store Write2 : DataStoreWrite  DataStoreName=LSO18_ETC_DC
  Data Store Write4 : DataStoreWrite  DataStoreName=LS012
  Data Store Write5 : DataStoreWrite  DataStoreName=LS013
  Data Store Write6 : DataStoreWrite  DataStoreName=LS002
  Data Store Write7 : DataStoreWrite  DataStoreName=LS004
  Data Store Write8 : DataStoreWrite  DataStoreName=LS009
  Data Store Write9 : DataStoreWrite  DataStoreName=LS011
  Data Type Conversion{,5..11} (8 alike) : DataTypeConversion  OutDataTypeStr=boolean
  Data Type Conversion{3..4,13..16} (6 alike) : DataTypeConversion
  Lv_to_Dut1 : Subsystem
  Lv_to_Dut2 : Subsystem
  Lv_to_Dut3 : Subsystem
  Max3 : MinMax  Function=max  Inputs=2
  ThermFR_RRvRead1 : Subsystem
  ThermFR_RRvRead2 : Subsystem
  ThermLvRead3 : Subsystem
  ACM_OUT : Outport
  wires:
  Bus Creator4/1 -> ACM_OUT/1
  BMS/1 -> Bus Selector/1
  RCU/1 -> Bus Selector1/1
  Data Type Conversion/1 -> Data Store Write/1
  ThermLvRead3/1(Fan_Low) -> Data Type Conversion5/1
  ThermLvRead3/6(v4) -> Data Type Conversion10/1
  ThermLvRead3/5(v3) -> Data Type Conversion9/1
  ThermLvRead3/4(v2) -> Data Type Conversion8/1
  ThermLvRead3/3(v1) -> Data Type Conversion7/1
  ThermLvRead3/2(Fan_High) -> Data Type Conversion6/1
  Bus Selector/1 -> Bus Creator4/1  "<BMS_PackMeasure>"
  ThermFR_RRvRead2/2(Fan_Low) -> Data Type Conversion/1
  ThermFR_RRvRead2/1(MtrPumpLvReq) -> Data Type Conversion3/1
  Lv_to_Dut1/1(MCUReqMtrPumpDut) -> Data Type Conversion4/1
  Bus Selector/2 -> Bus Creator4/2  "<BMS_PackStateInf>"
  Bus Selector1/1 -> Bus Creator4/3  "<RCU_GCUISGMotorActTemp>"
  Bus Selector1/2 -> Bus Creator4/4  "<RCU_EngCltTmp>"
  Bus Selector1/3 -> Bus Creator4/5  "<RCU_GCUISGInverterTempHiAlarm>"
  Data Type Conversion5/1 -> Data Store Write4/1
  Data Type Conversion6/1 -> Data Store Write5/1
  Data Type Conversion8/1 -> Data Store Write7/1
  Data Type Conversion7/1 -> Data Store Write6/1
  Data Type Conversion9/1 -> Data Store Write8/1
  Data Type Conversion10/1 -> Data Store Write9/1
  Data Type Conversion14/1 -> Data Store Write2/1
  Data Type Conversion13/1 -> Lv_to_Dut2/1(MCUReqMtrPumpLv)
  ThermFR_RRvRead1/2(Fan_Low) -> Data Type Conversion11/1
  ThermFR_RRvRead1/1(MtrPumpLvReq) -> Data Type Conversion13/1
  Data Store Read5/1 -> ThermLvRead3/1(RdySt), ThermFR_RRvRead1/1(RdySt), ThermFR_RRvRead2/1(RdySt)
  Lv_to_Dut2/1(MCUReqMtrPumpDut) -> Data Type Conversion14/1
  Data Type Conversion11/1 -> Data Store Write12/1
  Data Type Conversion16/1 -> Data Store Write10/1
  Lv_to_Dut3/1(MCUReqBatPumpDut) -> Data Type Conversion16/1
  ThermLvRead3/7(PumpLvReq) -> Data Type Conversion15/1
  Data Type Conversion15/1 -> Lv_to_Dut3/1(MCUReqBatPumpLv)
  Data Type Conversion4/1 -> Data Store Write14/1
  Data Type Conversion3/1 -> Lv_to_Dut1/1(MCUReqMtrPumpLv)
  DAQ/1 -> [DAQ]
  Bus Selector2/1 -> Max3/1  "<BatTempOut>"
  ptc/1 -> Bus Selector3/1
  Max3/1 -> ThermLvRead3/2(Temp)
  Bus Selector3/1 -> Max3/2  "<PTC_Coolanttemperature>"
  [DAQ] -> Bus Selector2/1
  [DAQ] -> Bus Selector5/1
  Bus Selector5/1 -> ThermFR_RRvRead2/2(MtrTemp)  "<MtrTempL>"
  Bus Selector4/1 -> ThermFR_RRvRead1/2(MtrTemp)  "<MtrTempR>"
  [DAQ] -> Bus Selector4/1

== system ZT_VehCtrl_18B/Initialization & SPI timer1/CS1 LS/Subsystem ==
  Data Store Read : DataStoreRead  DataStoreName=SPIO_CS1_InitFlg
  Merge : Merge  Inputs=3
  Merge1 : Merge  Inputs=3
  SPI_en : Subsystem  TreatAsAtomicUnit=on
  Switch Case : SwitchCase  CaseConditions={1,2,3}  ShowDefaultCase=off
  "clear " : Subsystem  TreatAsAtomicUnit=on
  confi_enbit : Subsystem  TreatAsAtomicUnit=on
  Out1 : Outport
  Out2 : Outport  Port=2
  wires:
  confi_enbit/1(Out1) -> Merge/3
  SPI_en/1(Out1) -> Merge/2
  "clear "/2(Out2) -> Merge1/1
  confi_enbit/2(Out2) -> Merge1/3
  "clear "/1(Out1) -> Merge/1
  Switch Case/1 -> "clear "/Action
  Switch Case/3 -> confi_enbit/Action
  Merge1/1 -> Out2/1
  Switch Case/2 -> SPI_en/Action
  SPI_en/2(Out2) -> Merge1/2
  Data Store Read/1 -> Switch Case/1
  Merge/1 -> Out1/1

== system ZT_VehCtrl_18B/Initialization & SPI timer1/CS3 LS/Subsystem ==
  In1 : Inport
  In2 : Inport  Port=2
  A组配置 : Subsystem  TreatAsAtomicUnit=on
  B组配置 : Subsystem  TreatAsAtomicUnit=on
  Data Store Read : DataStoreRead  DataStoreName=SPI3_CTRL1
  Merge : Merge  Inputs=3
  Merge1 : Merge  Inputs=3
  Switch Case : SwitchCase  CaseConditions={1,2,3}  ShowDefaultCase=off
  Out1 : Outport
  Out2 : Outport  Port=2
  Out3 : Outport  Port=3
  wires:
  Switch Case/2 -> B组配置/Action
  Merge1/1 -> Out3/1
  A组配置/2(Out2) -> Merge1/1
  In2/1 -> Merge1/3
  Data Store Read/1 -> Switch Case/1
  B组配置/1(Out1) -> Merge/2
  Merge/1 -> Out2/1
  Switch Case/3 -> Out1/1
  A组配置/1(Out1) -> Merge/1
  B组配置/2(Out2) -> Merge1/2
  Switch Case/1 -> A组配置/Action
  In1/1 -> Merge/3

== system ZT_VehCtrl_18B/Initialization & SPI timer1/CS5 LS/Subsystem ==
  Data Store Read : DataStoreRead  DataStoreName=SPIO_CS1_InitFlg
  Merge : Merge  Inputs=3
  Merge1 : Merge  Inputs=3
  SPI_en : Subsystem  TreatAsAtomicUnit=on
  Switch Case : SwitchCase  CaseConditions={1,2,3}  ShowDefaultCase=off
  "clear " : Subsystem  TreatAsAtomicUnit=on
  confi_enbit : Subsystem  TreatAsAtomicUnit=on
  Out1 : Outport
  Out2 : Outport  Port=2
  wires:
  confi_enbit/1(Out1) -> Merge/3
  SPI_en/1(Out1) -> Merge/2
  "clear "/2(Out2) -> Merge1/1
  confi_enbit/2(Out2) -> Merge1/3
  "clear "/1(Out1) -> Merge/1
  Switch Case/1 -> "clear "/Action
  Switch Case/3 -> confi_enbit/Action
  Merge1/1 -> Out2/1
  Switch Case/2 -> SPI_en/Action
  SPI_en/2(Out2) -> Merge1/2
  Data Store Read/1 -> Switch Case/1
  Merge/1 -> Out1/1

== system ZT_VehCtrl_18B/SPI_EEPROM/SPI_write/SPI_enable ==
  Action Port : ActionPort
  Constant1 : Constant  Value=2
  Data Store Write : DataStoreWrite  DataStoreName=Write_Ctrl
  Data Type Conversion : DataTypeConversion  OutDataTypeStr=uint8
  Data Type Conversion3 : DataTypeConversion
  Data Type Conversion8 : DataTypeConversion
  Demux1 : Demux  Outputs=1
  SPI_Master_Transfer_To1 : mbd_mpc574x_ec_toolbox/Communication Blocks/SPI Blocks/SPI_Master_Transfer  Priority=2  InstanceNumber=0  xfermode=Non blocking  timeout=50  spi_upd=on  WhichPCS=0
  Terminator : Terminator
  Vector Concatenate1 : Concatenate  NumInputs=1
  write_enable : Constant  Value=6  OutDataTypeStr=uint8
  wires:
  Data Type Conversion3/1 -> Terminator/1  "r8"
  SPI_Master_Transfer_To1/1 -> Demux1/1
  Demux1/1 -> Data Type Conversion3/1
  Vector Concatenate1/1 -> SPI_Master_Transfer_To1/1
  write_enable/1 -> Data Type Conversion/1
  Data Type Conversion/1 -> Vector Concatenate1/1  "d8"
  Constant1/1 -> Data Type Conversion8/1
  Data Type Conversion8/1 -> Data Store Write/1

== system ZT_VehCtrl_18B/SPI_EEPROM/SPI_write/SPI_write ==
  Action Port : ActionPort
  "Address_High " : Constant  Value=hex2dec('FF')  OutDataTypeStr=uint8
  Address_Low : Constant  Value=hex2dec('FF')
  Constant1 : Constant
  Data Store Read : DataStoreRead  DataStoreName=A_write
  Data Store Write : DataStoreWrite  DataStoreName=Write_Ctrl
  Data Type Conversion{,1..2,5} (4 alike) : DataTypeConversion  OutDataTypeStr=uint8
  Data Type Conversion{3..4,6..8} (5 alike) : DataTypeConversion
  Demux1 : Demux
  SPI_Master_Transfer_To1 : mbd_mpc574x_ec_toolbox/Communication Blocks/SPI Blocks/SPI_Master_Transfer  Priority=2  InstanceNumber=0  xfermode=Non blocking  timeout=50  spi_upd=on  WhichPCS=0
  Terminator{,1..3} (4 alike) : Terminator
  Vector Concatenate1 : Concatenate  NumInputs=4
  write_set : Constant  Value=2  OutDataTypeStr=uint8
  wires:
  Data Type Conversion4/1 -> Terminator1/1  "r5"
  Data Type Conversion3/1 -> Terminator/1  "r4"
  SPI_Master_Transfer_To1/1 -> Demux1/1
  Demux1/1 -> Data Type Conversion3/1
  Vector Concatenate1/1 -> SPI_Master_Transfer_To1/1
  Demux1/2 -> Data Type Conversion4/1
  Address_Low/1 -> Data Type Conversion5/1
  Data Type Conversion/1 -> Vector Concatenate1/1  "d4"
  Data Type Conversion1/1 -> Vector Concatenate1/2  "d5"
  write_set/1 -> Data Type Conversion/1
  "Address_High "/1 -> Data Type Conversion1/1
  Data Store Read/1 -> Data Type Conversion2/1
  Constant1/1 -> Data Type Conversion8/1
  Data Type Conversion5/1 -> Vector Concatenate1/3  "d6"
  Data Type Conversion2/1 -> Vector Concatenate1/4  "d7"
  Data Type Conversion6/1 -> Terminator2/1  "r6"
  Demux1/3 -> Data Type Conversion6/1
  Data Type Conversion7/1 -> Terminator3/1  "r7"
  Demux1/4 -> Data Type Conversion7/1
  Data Type Conversion8/1 -> Data Store Write/1

== system ZT_VehCtrl_18B/SigIn/CAN0 /BMS Cell Battery Temperature ==
  ID : Inport
  Data : Inport  Port=2
  length : Inport  Port=3
  timestamp : Inport  Port=4
  Switch Case : SwitchCase  CaseConditions={hex2dec('357')}  ShowDefaultCase=off
  UNPACK : Subsystem  TreatAsAtomicUnit=on
  Message : Outport
  wires:
  UNPACK/1(Message) -> Message/1
  length/1 -> UNPACK/3(length)
  timestamp/1 -> UNPACK/4(timestamp)
  Data/1 -> UNPACK/2(data)
  ID/1 -> Switch Case/1, UNPACK/1(ID)
  Switch Case/1 -> UNPACK/Action

== system ZT_VehCtrl_18B/SigIn/CAN0 /BMS Cell HeatingTemperature ==
  ID : Inport
  Data : Inport  Port=2
  length : Inport  Port=3
  timestamp : Inport  Port=4
  Switch Case : SwitchCase  CaseConditions={hex2dec('3F3')}  ShowDefaultCase=off
  UNPACK : Subsystem  TreatAsAtomicUnit=on
  Message : Outport
  wires:
  Switch Case/1 -> UNPACK/Action
  ID/1 -> UNPACK/1(ID), Switch Case/1
  Data/1 -> UNPACK/2(data)
  timestamp/1 -> UNPACK/4(timestamp)
  length/1 -> UNPACK/3(length)
  UNPACK/1(Message) -> Message/1

== system ZT_VehCtrl_18B/SigIn/CAN0 /BMS Cell Pole Temperature ==
  ID : Inport
  Data : Inport  Port=2
  length : Inport  Port=3
  timestamp : Inport  Port=4
  Switch Case : SwitchCase  CaseConditions={hex2dec('3F4')}  ShowDefaultCase=off
  UNPACK : Subsystem  TreatAsAtomicUnit=on
  Message : Outport
  wires:
  UNPACK/1(Message) -> Message/1
  length/1 -> UNPACK/3(length)
  timestamp/1 -> UNPACK/4(timestamp)
  Data/1 -> UNPACK/2(data)
  ID/1 -> Switch Case/1, UNPACK/1(ID)
  Switch Case/1 -> UNPACK/Action

== system ZT_VehCtrl_18B/SigIn/CAN0 /BMS Cell Voltage Infor ==
  ID : Inport
  Data : Inport  Port=2
  length : Inport  Port=3
  timestamp : Inport  Port=4
  Switch Case : SwitchCase  CaseConditions={hex2dec('356')}  ShowDefaultCase=off
  UNPACK : Subsystem  TreatAsAtomicUnit=on
  Message : Outport
  wires:
  UNPACK/1(Message) -> Message/1
  length/1 -> UNPACK/3(length)
  timestamp/1 -> UNPACK/4(timestamp)
  Data/1 -> UNPACK/2(data)
  ID/1 -> Switch Case/1, UNPACK/1(ID)
  Switch Case/1 -> UNPACK/Action

== system ZT_VehCtrl_18B/SigIn/CAN0 /BMS CumuCap Infor ==
  ID : Inport
  Data : Inport  Port=2
  length : Inport  Port=3
  timestamp : Inport  Port=4
  Switch Case : SwitchCase  CaseConditions={hex2dec('3F5')}  ShowDefaultCase=off
  UNPACK : Subsystem  TreatAsAtomicUnit=on
  Message : Outport
  wires:
  Switch Case/1 -> UNPACK/Action
  ID/1 -> UNPACK/1(ID), Switch Case/1
  Data/1 -> UNPACK/2(data)
  timestamp/1 -> UNPACK/4(timestamp)
  length/1 -> UNPACK/3(length)
  UNPACK/1(Message) -> Message/1

== system ZT_VehCtrl_18B/SigIn/CAN0 /BMS CumuTimeInfor1 ==
  ID : Inport
  Data : Inport  Port=2
  length : Inport  Port=3
  timestamp : Inport  Port=4
  Switch Case : SwitchCase  CaseConditions={hex2dec('203')}  ShowDefaultCase=off
  UNPACK : Subsystem  TreatAsAtomicUnit=on
  Message : Outport
  wires:
  UNPACK/1(Message) -> Message/1
  length/1 -> UNPACK/3(length)
  timestamp/1 -> UNPACK/4(timestamp)
  Data/1 -> UNPACK/2(data)
  ID/1 -> Switch Case/1, UNPACK/1(ID)
  Switch Case/1 -> UNPACK/Action

== system ZT_VehCtrl_18B/SigIn/CAN0 /BMS CumuTimeInfor2 ==
  ID : Inport
  Data : Inport  Port=2
  length : Inport  Port=3
  timestamp : Inport  Port=4
  Switch Case : SwitchCase  CaseConditions={hex2dec('204')}  ShowDefaultCase=off
  UNPACK : Subsystem  TreatAsAtomicUnit=on
  Message : Outport
  wires:
  Switch Case/1 -> UNPACK/Action
  ID/1 -> UNPACK/1(ID), Switch Case/1
  Data/1 -> UNPACK/2(data)
  timestamp/1 -> UNPACK/4(timestamp)
  length/1 -> UNPACK/3(length)
  UNPACK/1(Message) -> Message/1

== system ZT_VehCtrl_18B/SigIn/CAN0 /BMS HeatInfor ==
  ID : Inport
  Data : Inport  Port=2
  length : Inport  Port=3
  timestamp : Inport  Port=4
  Switch Case : SwitchCase  CaseConditions={hex2dec('208')}  ShowDefaultCase=off
  UNPACK : Subsystem  TreatAsAtomicUnit=on
  Message : Outport
  wires:
  Switch Case/1 -> UNPACK/Action
  ID/1 -> UNPACK/1(ID), Switch Case/1
  Data/1 -> UNPACK/2(data)
  timestamp/1 -> UNPACK/4(timestamp)
  length/1 -> UNPACK/3(length)
  UNPACK/1(Message) -> Message/1

== system ZT_VehCtrl_18B/SigIn/CAN0 /BMS Power Control ==
  ID : Inport
  Data : Inport  Port=2
  length : Inport  Port=3
  timestamp : Inport  Port=4
  Switch Case : SwitchCase  CaseConditions={hex2dec('1F3')}  ShowDefaultCase=off
  UNPACK : Subsystem  TreatAsAtomicUnit=on
  Message : Outport
  wires:
  Switch Case/1 -> UNPACK/Action
  ID/1 -> UNPACK/1(ID), Switch Case/1
  Data/1 -> UNPACK/2(data)
  timestamp/1 -> UNPACK/4(timestamp)
  length/1 -> UNPACK/3(length)
  UNPACK/1(Message) -> Message/1

== system ZT_VehCtrl_18B/SigIn/CAN0 /BMS Power Infor ==
  ID : Inport
  Data : Inport  Port=2
  length : Inport  Port=3
  timestamp : Inport  Port=4
  Switch Case : SwitchCase  CaseConditions={hex2dec('211')}  ShowDefaultCase=off
  UNPACK : Subsystem  TreatAsAtomicUnit=on
  Message : Outport
  wires:
  Switch Case/1 -> UNPACK/Action
  ID/1 -> UNPACK/1(ID), Switch Case/1
  Data/1 -> UNPACK/2(data)
  timestamp/1 -> UNPACK/4(timestamp)
  length/1 -> UNPACK/3(length)
  UNPACK/1(Message) -> Message/1

== system ZT_VehCtrl_18B/SigIn/CAN0 /BMS StartDia_Infor1 ==
  ID : Inport
  Data : Inport  Port=2
  length : Inport  Port=3
  timestamp : Inport  Port=4
  Switch Case : SwitchCase  CaseConditions={hex2dec('206')}  ShowDefaultCase=off
  UNPACK : Subsystem  TreatAsAtomicUnit=on
  Message : Outport
  wires:
  Switch Case/1 -> UNPACK/Action
  ID/1 -> UNPACK/1(ID), Switch Case/1
  Data/1 -> UNPACK/2(data)
  timestamp/1 -> UNPACK/4(timestamp)
  length/1 -> UNPACK/3(length)
  UNPACK/1(Message) -> Message/1

== system ZT_VehCtrl_18B/SigIn/CAN0 /BMS StartDia_Infor2 ==
  ID : Inport
  Data : Inport  Port=2
  length : Inport  Port=3
  timestamp : Inport  Port=4
  Switch Case : SwitchCase  CaseConditions={hex2dec('207')}  ShowDefaultCase=off
  UNPACK : Subsystem  TreatAsAtomicUnit=on
  Message : Outport
  wires:
  UNPACK/1(Message) -> Message/1
  length/1 -> UNPACK/3(length)
  timestamp/1 -> UNPACK/4(timestamp)
  Data/1 -> UNPACK/2(data)
  ID/1 -> Switch Case/1, UNPACK/1(ID)
  Switch Case/1 -> UNPACK/Action

== system ZT_VehCtrl_18B/SigIn/CAN0 /BMS Statistic_Cell ExtremumIndex Infor ==
  ID : Inport
  Data : Inport  Port=2
  length : Inport  Port=3
  timestamp : Inport  Port=4
  Switch Case : SwitchCase  CaseConditions={hex2dec('358')}  ShowDefaultCase=off
  UNPACK : Subsystem  TreatAsAtomicUnit=on
  Message : Outport
  wires:
  UNPACK/1(Message) -> Message/1
  length/1 -> UNPACK/3(length)
  timestamp/1 -> UNPACK/4(timestamp)
  Data/1 -> UNPACK/2(data)
  ID/1 -> Switch Case/1, UNPACK/1(ID)
  Switch Case/1 -> UNPACK/Action

== system ZT_VehCtrl_18B/SigIn/CAN0 /BMS Statistic_Cell Voltage Infor ==
  ID : Inport
  Data : Inport  Port=2
  length : Inport  Port=3
  timestamp : Inport  Port=4
  Switch Case : SwitchCase  CaseConditions={hex2dec('352')}  ShowDefaultCase=off
  UNPACK : Subsystem  TreatAsAtomicUnit=on
  Message : Outport
  wires:
  UNPACK/1(Message) -> Message/1
  length/1 -> UNPACK/3(length)
  timestamp/1 -> UNPACK/4(timestamp)
  Data/1 -> UNPACK/2(data)
  ID/1 -> Switch Case/1, UNPACK/1(ID)
  Switch Case/1 -> UNPACK/Action

== system ZT_VehCtrl_18B/SigIn/CAN0 /BMS Statistic_HeatingTemperature ==
  ID : Inport
  Data : Inport  Port=2
  length : Inport  Port=3
  timestamp : Inport  Port=4
  Switch Case : SwitchCase  CaseConditions={hex2dec('354')}  ShowDefaultCase=off
  UNPACK : Subsystem  TreatAsAtomicUnit=on
  Message : Outport
  wires:
  UNPACK/1(Message) -> Message/1
  length/1 -> UNPACK/3(length)
  timestamp/1 -> UNPACK/4(timestamp)
  Data/1 -> UNPACK/2(data)
  ID/1 -> Switch Case/1, UNPACK/1(ID)
  Switch Case/1 -> UNPACK/Action

== system ZT_VehCtrl_18B/SigIn/CAN0 /BMS Statistic_PoleTemperature ==
  ID : Inport
  Data : Inport  Port=2
  length : Inport  Port=3
  timestamp : Inport  Port=4
  Switch Case : SwitchCase  CaseConditions={hex2dec('355')}  ShowDefaultCase=off
  UNPACK : Subsystem  TreatAsAtomicUnit=on
  Message : Outport
  wires:
  UNPACK/1(Message) -> Message/1
  length/1 -> UNPACK/3(length)
  timestamp/1 -> UNPACK/4(timestamp)
  Data/1 -> UNPACK/2(data)
  ID/1 -> Switch Case/1, UNPACK/1(ID)
  Switch Case/1 -> UNPACK/Action

== system ZT_VehCtrl_18B/SigIn/CAN0 /BMS Statistic_Temperature of Battery ==
  ID : Inport
  Data : Inport  Port=2
  length : Inport  Port=3
  timestamp : Inport  Port=4
  Switch Case : SwitchCase  CaseConditions={hex2dec('353')}  ShowDefaultCase=off
  UNPACK : Subsystem  TreatAsAtomicUnit=on
  Message : Outport
  wires:
  UNPACK/1(Message) -> Message/1
  length/1 -> UNPACK/3(length)
  timestamp/1 -> UNPACK/4(timestamp)
  Data/1 -> UNPACK/2(data)
  ID/1 -> Switch Case/1, UNPACK/1(ID)
  Switch Case/1 -> UNPACK/Action

== system ZT_VehCtrl_18B/SigIn/CAN0 /BMS _SystemTime  ==
  ID : Inport
  Data : Inport  Port=2
  length : Inport  Port=3
  timestamp : Inport  Port=4
  Switch Case : SwitchCase  CaseConditions={hex2dec('202')}  ShowDefaultCase=off
  UNPACK : Subsystem  TreatAsAtomicUnit=on
  Message : Outport
  wires:
  Switch Case/1 -> UNPACK/Action
  ID/1 -> UNPACK/1(ID), Switch Case/1
  Data/1 -> UNPACK/2(data)
  timestamp/1 -> UNPACK/4(timestamp)
  length/1 -> UNPACK/3(length)
  UNPACK/1(Message) -> Message/1

== system ZT_VehCtrl_18B/SigIn/CAN0 /BMS other Information1 ==
  ID : Inport
  Data : Inport  Port=2
  length : Inport  Port=3
  timestamp : Inport  Port=4
  Switch Case : SwitchCase  CaseConditions={hex2dec('3F6')}  ShowDefaultCase=off
  UNPACK : Subsystem  TreatAsAtomicUnit=on
  Message : Outport
  wires:
  UNPACK/1(Message) -> Message/1
  length/1 -> UNPACK/3(length)
  timestamp/1 -> UNPACK/4(timestamp)
  Data/1 -> UNPACK/2(data)
  ID/1 -> Switch Case/1, UNPACK/1(ID)
  Switch Case/1 -> UNPACK/Action

== system ZT_VehCtrl_18B/SigIn/CAN0 /BMS other Information2  ==
  ID : Inport
  Data : Inport  Port=2
  length : Inport  Port=3
  timestamp : Inport  Port=4
  Switch Case : SwitchCase  CaseConditions={hex2dec('3FF')}  ShowDefaultCase=off
  UNPACK : Subsystem  TreatAsAtomicUnit=on
  Message : Outport
  wires:
  Switch Case/1 -> UNPACK/Action
  ID/1 -> UNPACK/1(ID), Switch Case/1
  Data/1 -> UNPACK/2(data)
  timestamp/1 -> UNPACK/4(timestamp)
  length/1 -> UNPACK/3(length)
  UNPACK/1(Message) -> Message/1

== system ZT_VehCtrl_18B/SigIn/CAN0 /BMS other Information3 ==
  ID : Inport
  Data : Inport  Port=2
  length : Inport  Port=3
  timestamp : Inport  Port=4
  Switch Case : SwitchCase  CaseConditions={hex2dec('205')}  ShowDefaultCase=off
  UNPACK : Subsystem  TreatAsAtomicUnit=on
  Message : Outport
  wires:
  UNPACK/1(Message) -> Message/1
  length/1 -> UNPACK/3(length)
  timestamp/1 -> UNPACK/4(timestamp)
  Data/1 -> UNPACK/2(data)
  ID/1 -> Switch Case/1, UNPACK/1(ID)
  Switch Case/1 -> UNPACK/Action

== system ZT_VehCtrl_18B/SigIn/CAN0 /BMSWarning_Status ==
  ID : Inport
  Data : Inport  Port=2
  length : Inport  Port=3
  timestamp : Inport  Port=4
  Switch Case : SwitchCase  CaseConditions={hex2dec('1F5')}  ShowDefaultCase=off
  UNPACK : Subsystem  TreatAsAtomicUnit=on
  Message : Outport
  wires:
  UNPACK/1(Message) -> Message/1
  length/1 -> UNPACK/3(length)
  timestamp/1 -> UNPACK/4(timestamp)
  Data/1 -> UNPACK/2(data)
  ID/1 -> Switch Case/1, UNPACK/1(ID)
  Switch Case/1 -> UNPACK/Action

== system ZT_VehCtrl_18B/SigIn/CAN0 /BMS_Information1 ==
  ID : Inport
  Data : Inport  Port=2
  length : Inport  Port=3
  timestamp : Inport  Port=4
  Switch Case : SwitchCase  CaseConditions={hex2dec('1E1')}  ShowDefaultCase=off
  UNPACK : Subsystem  TreatAsAtomicUnit=on
  Message : Outport
  wires:
  UNPACK/1(Message) -> Message/1
  length/1 -> UNPACK/3(length)
  timestamp/1 -> UNPACK/4(timestamp)
  Data/1 -> UNPACK/2(data)
  ID/1 -> Switch Case/1, UNPACK/1(ID)
  Switch Case/1 -> UNPACK/Action

== system ZT_VehCtrl_18B/SigIn/CAN0 /BMS_Information2 ==
  ID : Inport
  Data : Inport  Port=2
  length : Inport  Port=3
  timestamp : Inport  Port=4
  Switch Case : SwitchCase  CaseConditions={hex2dec('1E4')}  ShowDefaultCase=off
  UNPACK : Subsystem  TreatAsAtomicUnit=on
  Message : Outport
  wires:
  Switch Case/1 -> UNPACK/Action
  ID/1 -> UNPACK/1(ID), Switch Case/1
  Data/1 -> UNPACK/2(data)
  timestamp/1 -> UNPACK/4(timestamp)
  length/1 -> UNPACK/3(length)
  UNPACK/1(Message) -> Message/1

== system ZT_VehCtrl_18B/SigIn/CAN0 /BMS_Relay Status ==
  ID : Inport
  Data : Inport  Port=2
  length : Inport  Port=3
  timestamp : Inport  Port=4
  Switch Case : SwitchCase  CaseConditions={hex2dec('351')}  ShowDefaultCase=off
  UNPACK : Subsystem  TreatAsAtomicUnit=on
  Message : Outport
  wires:
  UNPACK/1(Message) -> Message/1
  length/1 -> UNPACK/3(length)
  timestamp/1 -> UNPACK/4(timestamp)
  Data/1 -> UNPACK/2(data)
  ID/1 -> Switch Case/1, UNPACK/1(ID)
  Switch Case/1 -> UNPACK/Action

== system ZT_VehCtrl_18B/SigIn/CAN0 /BMS_Relay Status2 ==
  ID : Inport
  Data : Inport  Port=2
  length : Inport  Port=3
  timestamp : Inport  Port=4
  Switch Case : SwitchCase  CaseConditions={hex2dec('360')}  ShowDefaultCase=off
  UNPACK : Subsystem  TreatAsAtomicUnit=on
  Message : Outport
  wires:
  UNPACK/1(Message) -> Message/1
  length/1 -> UNPACK/3(length)
  timestamp/1 -> UNPACK/4(timestamp)
  Data/1 -> UNPACK/2(data)
  ID/1 -> Switch Case/1, UNPACK/1(ID)
  Switch Case/1 -> UNPACK/Action

== system ZT_VehCtrl_18B/SigIn/CAN0 /BMS_Relay Status3 ==
  ID : Inport
  Data : Inport  Port=2
  length : Inport  Port=3
  timestamp : Inport  Port=4
  Switch Case : SwitchCase  CaseConditions={hex2dec('361')}  ShowDefaultCase=off
  UNPACK : Subsystem  TreatAsAtomicUnit=on
  Message : Outport
  wires:
  Switch Case/1 -> UNPACK/Action
  ID/1 -> UNPACK/1(ID), Switch Case/1
  Data/1 -> UNPACK/2(data)
  timestamp/1 -> UNPACK/4(timestamp)
  length/1 -> UNPACK/3(length)
  UNPACK/1(Message) -> Message/1

== system ZT_VehCtrl_18B/SigIn/CAN0 /BRS2VCU1 ==
  ID : Inport
  Data : Inport  Port=2
  length : Inport  Port=3
  timestamp : Inport  Port=4
  Switch Case : SwitchCase  CaseConditions={hex2dec('18FE25E4')}  ShowDefaultCase=off
  UNPACK : Subsystem  TreatAsAtomicUnit=on
  Message : Outport
  wires:
  Switch Case/1 -> UNPACK/Action
  ID/1 -> UNPACK/1(ID), Switch Case/1
  Data/1 -> UNPACK/2(data)
  timestamp/1 -> UNPACK/4(timestamp)
  length/1 -> UNPACK/3(length)
  UNPACK/1(Message) -> Message/1

== system ZT_VehCtrl_18B/SigIn/CAN0 /BRS2VCU2 ==
  ID : Inport
  Data : Inport  Port=2
  length : Inport  Port=3
  timestamp : Inport  Port=4
  Switch Case : SwitchCase  CaseConditions={hex2dec('18FE26E4')}  ShowDefaultCase=off
  UNPACK : Subsystem  TreatAsAtomicUnit=on
  Message : Outport
  wires:
  UNPACK/1(Message) -> Message/1
  length/1 -> UNPACK/3(length)
  timestamp/1 -> UNPACK/4(timestamp)
  Data/1 -> UNPACK/2(data)
  ID/1 -> Switch Case/1, UNPACK/1(ID)
  Switch Case/1 -> UNPACK/Action

== system ZT_VehCtrl_18B/SigIn/CAN0 /BRS2VCU3 ==
  ID : Inport
  Data : Inport  Port=2
  length : Inport  Port=3
  timestamp : Inport  Port=4
  Switch Case : SwitchCase  CaseConditions={hex2dec('18FE27E4')}  ShowDefaultCase=off
  UNPACK : Subsystem  TreatAsAtomicUnit=on
  Message : Outport
  wires:
  Switch Case/1 -> UNPACK/Action
  ID/1 -> UNPACK/1(ID), Switch Case/1
  Data/1 -> UNPACK/2(data)
  timestamp/1 -> UNPACK/4(timestamp)
  length/1 -> UNPACK/3(length)
  UNPACK/1(Message) -> Message/1

== system ZT_VehCtrl_18B/SigIn/CAN0 /OBC_Charger Status ==
  ID : Inport
  Data : Inport  Port=2
  length : Inport  Port=3
  timestamp : Inport  Port=4
  Switch Case : SwitchCase  CaseConditions={hex2dec('220')}  ShowDefaultCase=off
  UNPACK : Subsystem  TreatAsAtomicUnit=on
  Message : Outport
  wires:
  Switch Case/1 -> UNPACK/Action
  ID/1 -> UNPACK/1(ID), Switch Case/1
  Data/1 -> UNPACK/2(data)
  timestamp/1 -> UNPACK/4(timestamp)
  length/1 -> UNPACK/3(length)
  UNPACK/1(Message) -> Message/1

== system ZT_VehCtrl_18B/SigIn/CAN0 /TMS2VCU ==
  ID : Inport
  Data : Inport  Port=2
  length : Inport  Port=3
  timestamp : Inport  Port=4
  Switch Case : SwitchCase  CaseConditions={hex2dec('18FFF346')}  ShowDefaultCase=off
  UNPACK : Subsystem  TreatAsAtomicUnit=on
  Message : Outport
  wires:
  UNPACK/1(Message) -> Message/1
  length/1 -> UNPACK/3(length)
  timestamp/1 -> UNPACK/4(timestamp)
  Data/1 -> UNPACK/2(data)
  ID/1 -> Switch Case/1, UNPACK/1(ID)
  Switch Case/1 -> UNPACK/Action
